simulink model "mrac_model"  (R2022a)
settings: Solver=VariableStepAuto  StartTime=0.0  StopTime=100  RelTol=1e-3
values from neighbouring files (symbols this model uses):
  params = getParamsMRAC(0.25, 1, 10e-3, 10e-5, 100)    [mrac.m]
libraries: slctrlblks x1
settings Model: Creator=mateusz  LastModifiedBy=mateusz

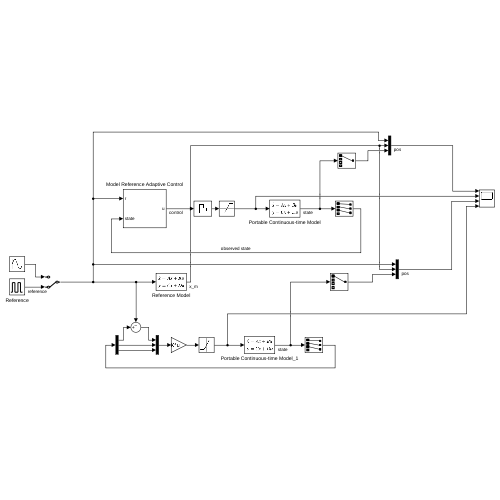
[thumbnail: Simulink's stored preview of the top-level diagram]
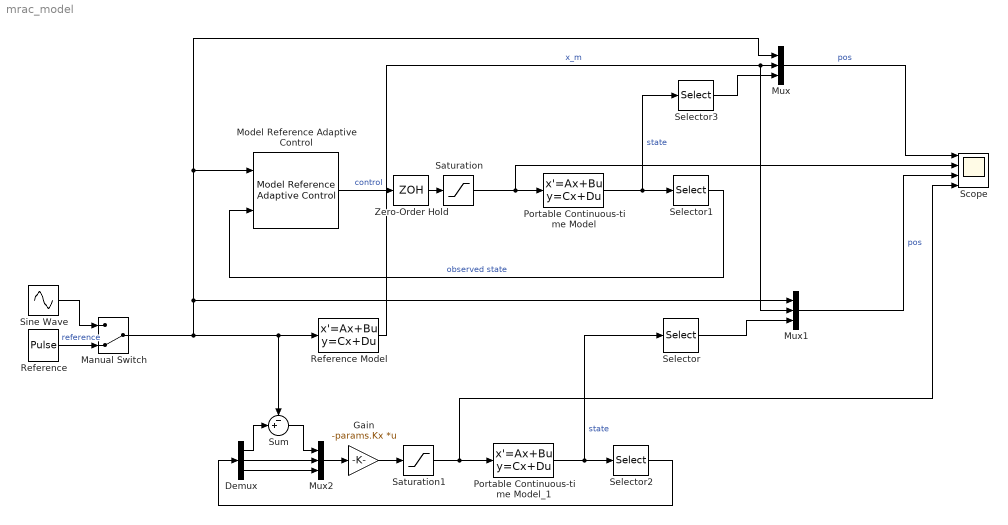
== system mrac_model ==
  Demux : Demux  Outputs=3
  Gain : Gain  Gain=-params.Kx  Multiplication=Matrix(K*u)
  Manual Switch : ManualSwitch  CurrentSetting=0
  Model Reference Adaptive Control : slctrlblks/Model Reference Adaptive Control  selectType=Direct  A=params.A - params.B*params.Kx  B=params.B*params.Kx(1)  Ahat=0  ALrEnable=on  gamma_a=1  ALrEnableMod=on  Bhat=1  BLrEnable=on  gamma_b=1  BLrEnableMod=on  externalKtauEnable=off  k_tau=-1  estParamOutput=off  Am=params.A - params.B*params.Kx  Bm=params.B*params.Kx(1)  kx=-params.Kx  FBLrEnable=on  gamma_kx=params.gamma_x  FBLrEnableMod=off  kr=params.Kr  FFLrEnable=off  gamma_kr=0.001  FFLrEnableMod=off  AdaptEnable=on  gamma=params.gamma_w  WLrEnableMod=off  Q=max(max(params.Q))  FeatureTypeOptions=Radial Basis Function  nCen=4  cSpanMin=-1  cSpanMax=1  cSig=5  adaptiveCntrlOutport=off  modChoice=None  sigma_val=0.1
      settings: SourceProductBaseCode=SD
  Mux : Mux  Inputs=3
  Mux1 : Mux  Inputs=3
  Mux2 : Mux  Inputs=3
  Portable Continuous-time Model : StateSpace  A=|  B=[0;0;0;2.59e4];  C=eye(4,4)  D=zeros(4,1)  InitialCondition=0
      | [0  1  0    0;
      |      0 -5  4.5  0;
      |      0  0 -0.7108*2  2*23.6012;
      |      0  0 -5.3898 -4040];
  Portable Continuous-time Model_1 : StateSpace  A=|  B=[0;0;0;2.59e4];  C=eye(4,4)  D=zeros(4,1)  InitialCondition=0
      | [0  1  0    0;
      |      0 -5  4.5  0;
      |      0  0 -0.7108*2  2*23.6012;
      |      0  0 -5.3898 -4040];
  Reference : DiscretePulseGenerator  PulseType=Time based  Amplitude=100  Period=50  PulseWidth=50
  Reference Model : StateSpace  A=params.A - params.B*params.Kx  B=params.B * params.Kx(1)  C=[1 0 0]  D=0  InitialCondition=0
  Saturation : Saturate  UpperLimit=1  LowerLimit=-1
  Saturation1 : Saturate  UpperLimit=1  LowerLimit=-1
  Scope : Scope  NumInputPorts=4
  Selector : Selector  InputPortWidth=4  IndexOptions=Index vector (dialog)  Indices=[1]  OutputSizes=1
  Selector1 : Selector  InputPortWidth=4  IndexOptions=Index vector (dialog)  Indices=[1 2 3]  OutputSizes=1
  Selector2 : Selector  InputPortWidth=4  IndexOptions=Index vector (dialog)  Indices=[1 2 3]  OutputSizes=1
  Selector3 : Selector  InputPortWidth=4  IndexOptions=Index vector (dialog)  Indices=[1]  OutputSizes=1
  Sine Wave : Sin  Amplitude=100  SampleTime=0
  Sum : Sum  Inputs=-+|
  Zero-Order Hold : ZeroOrderHold  SampleTime=0.01
  wires:
  Portable Continuous-time Model/1 -> Selector1/1, Selector3/1  "state"
  Selector1/1 -> Model Reference Adaptive Control/2  "observed state"
  Model Reference Adaptive Control/1 -> Zero-Order Hold/1  "control"
  Selector3/1 -> Mux/3
  Reference Model/1 -> Mux1/2, Mux/2  "x_m"
  Mux/1 -> Scope/1  "pos"
  Portable Continuous-time Model_1/1 -> Selector/1, Selector2/1  "state"
  Selector/1 -> Mux1/3
  Mux1/1 -> Scope/3  "pos"
  Gain/1 -> Saturation1/1
  Mux2/1 -> Gain/1
  Sum/1 -> Mux2/1
  Selector2/1 -> Demux/1
  Demux/1 -> Sum/2
  Demux/2 -> Mux2/2
  Demux/3 -> Mux2/3
  Saturation1/1 -> Scope/4, Portable Continuous-time Model_1/1
  Manual Switch/1 -> Reference Model/1, Sum/1, Mux/1, Model Reference Adaptive Control/1, Mux1/1
  Sine Wave/1 -> Manual Switch/1
  Reference/1 -> Manual Switch/2  "reference"
  Saturation/1 -> Scope/2, Portable Continuous-time Model/1
  Zero-Order Hold/1 -> Saturation/1
